simulink library "LiBatteryElements_backup_lib"  (R2020b)
settings: Solver=VariableStepAuto  StartTime=0.0  StopTime=10.0  RelTol=1e-3
values from neighbouring files (symbols this model uses):
  Q = capacity*3600*num_cells    [main.m]    (also in main_1S2P.m; main_cell.m = 4.6)
  SOC_0 = 1    [main.m]    (also in main_1S2P.m; main_cell.m)
undefined symbols (not defined in the file or in its folder): gcbh, simscape, T_init
libraries: fl_lib x10, $bdroot x4
settings Model: Creator=Vivian  LastModifiedBy=Vivian

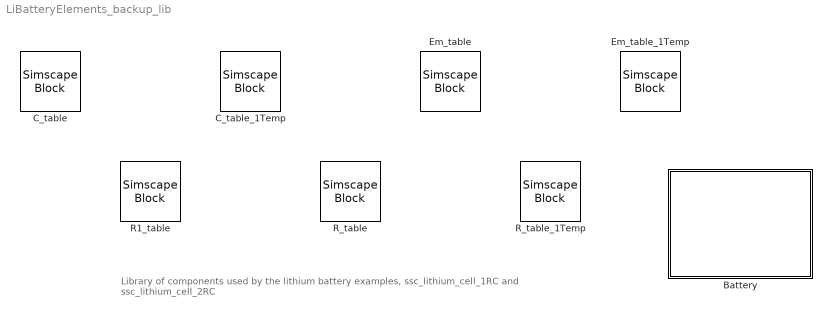
== system LiBatteryElements_backup_lib ==
  note: Library of components used by the lithium battery examples, ssc_lithium_cell_1RC and ssc_lithium_cell_2RC
  Battery : Subsystem
  C_table : SimscapeBlock  DialogController=NetworkEngine.DynNeDlgSource  LoadFcn=simscape.compiler.sli.internal.callback('LoadFcn',gcbh);  SourceFile=LiBatteryElements.C_table  mask(C_table){ComponentPath=LiBatteryElements.C_table, ComponentVariants=["LiBatteryElements.C_table"], ComponentVariantNames=["C_table"], ClassName=C_table, SchemaVersion=1, C_Table=ones(5, 3), C_Table_unit=F, C_Table_conf=compiletime, SOC_Table=[0; .1; .5; .9; 1], SOC_Table_unit=1, SOC_Table_conf=compiletime, Temp_Table=[273.15, 293.15, 313.15], Temp_Table_unit=K, Temp_Table_conf=compiletime, v0=0, v0_unit=V, v0_conf=compiletime}
      mask prompts: C_Table "Matrix of capacitance values, C(SOC,T)"; SOC_Table "State of charge (SOC) breakpoints"; Temp_Table "Temperature (T) breakpoints"; v0 "Initial voltage across capacitor"
      mask help: Models a capacitor where the capacitance value (C) depends on an external physical signal inputs SOC and T. It is assumed that the capacitance value is slowly varying with time, and hence the equation i = C*dv/dt holds.
      mask init:
      | simscape.compiler.sli.internal.preinitmask(gcb);
      settings: CopyFcn=simscape.compiler.sli.internal.callback('CopyFcn',gcbh);  DeleteFcn=simscape.compiler.sli.internal.callback('DeleteFcn',gcbh);  ModelCloseFcn=simscape.compiler.sli.internal.callback('ModelCloseFcn',gcbh);  PreSaveFcn=simscape.compiler.sli.internal.callback('PreSaveFcn',gcbh);  PostSaveFcn=simscape.compiler.sli.internal.callback('PostSaveFcn',gcbh);  PreCopyFcn=simscape.compiler.sli.internal.callback('PreCopyFcn',gcbh);  PreDeleteFcn=simscape.compiler.sli.internal.callback('PreDeleteFcn',gcbh);  InternalSimscapePortConfiguration="{\"Bottom\":[],\"Left\":[{\"id\":\"p\",\"label\":\"+\",\"type\":\"foundation.electrical.electrical\"},{\"id\":\"T\",\"label\":\"T\",\"type\":\"input\"},{\"id\":\"SOC\",\"label\":\"SOC\",\"type\":\"input\"}],\"Right\":[{\"id\":\"n\",\"label\":\"-\",\"type\":\"foundation.electrical.electrical\"}],\"Top\":[]}"
      mask Help: web(nesl_help(gcbh))
      mask TypeOptions C_Table_unit: F | pF | nF | uF | mF
      mask TypeOptions C_Table_conf: compiletime | runtime
      mask TypeOptions SOC_Table_unit: 1
      mask TypeOptions SOC_Table_conf: compiletime | runtime
      mask TypeOptions Temp_Table_unit: K | degC | degF | degR | deltaK | deltadegC | deltadegF | deltadegR
      mask TypeOptions Temp_Table_conf: compiletime | runtime
      mask TypeOptions v0_unit: V | mV | kV
      mask TypeOptions v0_conf: compiletime | runtime
  C_table_1Temp : SimscapeBlock  DialogController=NetworkEngine.DynNeDlgSource  LoadFcn=simscape.compiler.sli.internal.callback('LoadFcn',gcbh);  SourceFile=LiBatteryElements.C_table_1Temp  mask(C_table_1Temp){ComponentPath=LiBatteryElements.C_table_1Temp, ComponentVariants=["LiBatteryElements.C_table_1Temp"], ComponentVariantNames=["C_table_1Temp"], ClassName=C_table_1Temp, SchemaVersion=1, C_Table=ones(5, 1), C_Table_unit=F, C_Table_conf=compiletime, SOC_Table=[0; .1; .5; .9; 1], SOC_Table_unit=1, SOC_Table_conf=compiletime, v0=0, v0_unit=V, v0_conf=compiletime}
      mask prompts: C_Table "Vector of capacitance values"; SOC_Table "Corresponding SOC breakpoints"; v0 "Initial voltage across capacitor"
      mask help: Models a capacitor where the capacitance value (C) depends on an external physical signal input SOC. It is assumed that the capacitance value is slowly varying with time, and hence the equation i = C*dv/dt holds.
      mask init:
      | simscape.compiler.sli.internal.preinitmask(gcb);
      settings: CopyFcn=simscape.compiler.sli.internal.callback('CopyFcn',gcbh);  DeleteFcn=simscape.compiler.sli.internal.callback('DeleteFcn',gcbh);  ModelCloseFcn=simscape.compiler.sli.internal.callback('ModelCloseFcn',gcbh);  PreSaveFcn=simscape.compiler.sli.internal.callback('PreSaveFcn',gcbh);  PostSaveFcn=simscape.compiler.sli.internal.callback('PostSaveFcn',gcbh);  PreCopyFcn=simscape.compiler.sli.internal.callback('PreCopyFcn',gcbh);  PreDeleteFcn=simscape.compiler.sli.internal.callback('PreDeleteFcn',gcbh);  InternalSimscapePortConfiguration="{\"Bottom\":[],\"Left\":[{\"id\":\"p\",\"label\":\"+\",\"type\":\"foundation.electrical.electrical\"},{\"id\":\"SOC\",\"label\":\"SOC\",\"type\":\"input\"}],\"Right\":[{\"id\":\"n\",\"label\":\"-\",\"type\":\"foundation.electrical.electrical\"}],\"Top\":[]}"
      mask Help: web(nesl_help(gcbh))
      mask TypeOptions C_Table_unit: F | pF | nF | uF | mF
      mask TypeOptions C_Table_conf: compiletime | runtime
      mask TypeOptions SOC_Table_unit: 1
      mask TypeOptions SOC_Table_conf: compiletime | runtime
      mask TypeOptions v0_unit: V | mV | kV
      mask TypeOptions v0_conf: compiletime | runtime
  Em_table : SimscapeBlock  DialogController=NetworkEngine.DynNeDlgSource  LoadFcn=simscape.compiler.sli.internal.callback('LoadFcn',gcbh);  SourceFile=LiBatteryElements.Em_table  mask(Em_table){ComponentPath=LiBatteryElements.Em_table, ComponentVariants=["LiBatteryElements.Em_table"], ComponentVariantNames=["Em_table"], ClassName=Em_table, SchemaVersion=1, C_Table=[29, 30, 31], C_Table_unit=hr*A, C_Table_conf=compiletime, Em_Table=3.8 * ones(5, 3), Em_Table_unit=V, Em_Table_conf=compiletime, SOC_Table=[0; .1; .5; .9; 1], SOC_Table_unit=1, SOC_Table_conf=compiletime, Temp_Table=[273.15, 293.15, 313.15], Temp_Table_unit=K, Temp_Table_conf=compiletime, Qinit=0, Qinit_unit=hr*A, Qinit_conf=compiletime}
      mask prompts: C_Table "Capacity values at specified temperature breakpoints"; Em_Table "Matrix of voltage values, Em(SOC,T)"; SOC_Table "State of charge (SOC) breakpoints"; Temp_Table "Temperature (T) breakpoints"; Qinit "Initial charge deficit"
      mask help: This block implements the cell's main branch voltage source, and determines values for capacity (C) and state of charge (SOC). The defining equations depend on cell temperature, T.
      mask init:
      | simscape.compiler.sli.internal.preinitmask(gcb);
      settings: CopyFcn=simscape.compiler.sli.internal.callback('CopyFcn',gcbh);  DeleteFcn=simscape.compiler.sli.internal.callback('DeleteFcn',gcbh);  ModelCloseFcn=simscape.compiler.sli.internal.callback('ModelCloseFcn',gcbh);  PreSaveFcn=simscape.compiler.sli.internal.callback('PreSaveFcn',gcbh);  PostSaveFcn=simscape.compiler.sli.internal.callback('PostSaveFcn',gcbh);  PreCopyFcn=simscape.compiler.sli.internal.callback('PreCopyFcn',gcbh);  PreDeleteFcn=simscape.compiler.sli.internal.callback('PreDeleteFcn',gcbh);  InternalSimscapePortConfiguration="{\"Bottom\":[],\"Left\":[{\"id\":\"p\",\"label\":\"+\",\"type\":\"foundation.electrical.electrical\"},{\"id\":\"C\",\"label\":\"C\",\"type\":\"output\"},{\"id\":\"SOC\",\"label\":\"SOC\",\"type\":\"output\"}],\"Right\":[{\"id\":\"n\",\"label\":\"-\",\"type\":\"foundation.electrical.electrical\"},{\"id\":\"T\",\"label\":\"T\",\"type\":\"input\"}],\"Top\":[]}"
      mask Help: web(nesl_help(gcbh))
      mask TypeOptions C_Table_unit: C | hr*A
      mask TypeOptions C_Table_conf: compiletime | runtime
      mask TypeOptions Em_Table_unit: V | mV | kV
      mask TypeOptions Em_Table_conf: compiletime | runtime
      mask TypeOptions SOC_Table_unit: 1
      mask TypeOptions SOC_Table_conf: compiletime | runtime
      mask TypeOptions Temp_Table_unit: K | degC | degF | degR | deltaK | deltadegC | deltadegF | deltadegR
      mask TypeOptions Temp_Table_conf: compiletime | runtime
      mask TypeOptions Qinit_unit: C | hr*A
      mask TypeOptions Qinit_conf: compiletime | runtime
  Em_table_1Temp : SimscapeBlock  DialogController=NetworkEngine.DynNeDlgSource  LoadFcn=simscape.compiler.sli.internal.callback('LoadFcn',gcbh);  SourceFile=LiBatteryElements.Em_table_1Temp  mask(Em_table_1Temp){ComponentPath=LiBatteryElements.Em_table_1Temp, ComponentVariants=["LiBatteryElements.Em_table_1Temp"], ComponentVariantNames=["Em_table_1Temp"], ClassName=Em_table_1Temp, SchemaVersion=1, Em_Table=3.8 * ones(5, 1), Em_Table_unit=V, Em_Table_conf=compiletime, SOC_Table=[0; .1; .5; .9; 1], SOC_Table_unit=1, SOC_Table_conf=compiletime, C=30, C_unit=hr*A, C_conf=compiletime, Qinit=0, Qinit_unit=hr*A, Qinit_conf=compiletime}
      mask prompts: Em_Table "Vector of voltage values, Em"; SOC_Table "Corresponding SOC breakpoints"; C "Capacity (scalar)"; Qinit "Initial charge deficit"
      mask help: This block implements the main branch voltage source, capacity, and state of charge (SOC). The defining equations are assumed not to depend on temperature.
      mask init:
      | simscape.compiler.sli.internal.preinitmask(gcb);
      settings: CopyFcn=simscape.compiler.sli.internal.callback('CopyFcn',gcbh);  DeleteFcn=simscape.compiler.sli.internal.callback('DeleteFcn',gcbh);  ModelCloseFcn=simscape.compiler.sli.internal.callback('ModelCloseFcn',gcbh);  PreSaveFcn=simscape.compiler.sli.internal.callback('PreSaveFcn',gcbh);  PostSaveFcn=simscape.compiler.sli.internal.callback('PostSaveFcn',gcbh);  PreCopyFcn=simscape.compiler.sli.internal.callback('PreCopyFcn',gcbh);  PreDeleteFcn=simscape.compiler.sli.internal.callback('PreDeleteFcn',gcbh);  InternalSimscapePortConfiguration="{\"Bottom\":[],\"Left\":[{\"id\":\"p\",\"label\":\"+\",\"type\":\"foundation.electrical.electrical\"},{\"id\":\"SOC\",\"label\":\"SOC\",\"type\":\"output\"}],\"Right\":[{\"id\":\"n\",\"label\":\"-\",\"type\":\"foundation.electrical.electrical\"}],\"Top\":[]}"
      mask Help: web(nesl_help(gcbh))
      mask TypeOptions Em_Table_unit: V | mV | kV
      mask TypeOptions Em_Table_conf: compiletime | runtime
      mask TypeOptions SOC_Table_unit: 1
      mask TypeOptions SOC_Table_conf: compiletime | runtime
      mask TypeOptions C_unit: C | hr*A
      mask TypeOptions C_conf: compiletime | runtime
      mask TypeOptions Qinit_unit: C | hr*A
      mask TypeOptions Qinit_conf: compiletime | runtime
  R1_table : SimscapeBlock  DialogController=NetworkEngine.DynNeDlgSource  LoadFcn=simscape.compiler.sli.internal.callback('LoadFcn',gcbh);  SourceFile=LiBatteryElements.R1_table  mask(R1_table){ComponentPath=LiBatteryElements.R1_table, ComponentVariants=["LiBatteryElements.R1_table"], ComponentVariantNames=["R1_table"], ClassName=R1_table, SchemaVersion=1, R_Table=1e-3 * ones(5, 3), R_Table_unit=Ohm, R_Table_conf=compiletime, SOC_Table=[0; .1; .5; .9; 1], SOC_Table_unit=1, SOC_Table_conf=compiletime, Temp_Table=[273.15, 293.15, 313.15], Temp_Table_unit=K, Temp_Table_conf=compiletime}
      mask prompts: R_Table "Matrix of resistance values, R(SOC,T)"; SOC_Table "State of charge (SOC) breakpoints"; Temp_Table "Temperature (T) breakpoints"
      mask help: Models a resistor where the resistance value (R) depends on an external physical signal inputs SOC and T.
      mask init:
      | simscape.compiler.sli.internal.preinitmask(gcb);
      settings: CopyFcn=simscape.compiler.sli.internal.callback('CopyFcn',gcbh);  DeleteFcn=simscape.compiler.sli.internal.callback('DeleteFcn',gcbh);  ModelCloseFcn=simscape.compiler.sli.internal.callback('ModelCloseFcn',gcbh);  PreSaveFcn=simscape.compiler.sli.internal.callback('PreSaveFcn',gcbh);  PostSaveFcn=simscape.compiler.sli.internal.callback('PostSaveFcn',gcbh);  PreCopyFcn=simscape.compiler.sli.internal.callback('PreCopyFcn',gcbh);  PreDeleteFcn=simscape.compiler.sli.internal.callback('PreDeleteFcn',gcbh);  InternalSimscapePortConfiguration="{\"Bottom\":[],\"Left\":[{\"id\":\"p\",\"label\":\"+\",\"type\":\"foundation.electrical.electrical\"},{\"id\":\"T\",\"label\":\"T\",\"type\":\"input\"},{\"id\":\"SOC\",\"label\":\"SOC\",\"type\":\"input\"}],\"Right\":[{\"id\":\"n\",\"label\":\"-\",\"type\":\"foundation.electrical.electrical\"},{\"id\":\"pow\",\"label\":\"POW\",\"type\":\"output\"}],\"Top\":[]}"
      mask Help: web(nesl_help(gcbh))
      mask TypeOptions R_Table_unit: Ohm | kOhm | MOhm | GOhm
      mask TypeOptions R_Table_conf: compiletime | runtime
      mask TypeOptions SOC_Table_unit: 1
      mask TypeOptions SOC_Table_conf: compiletime | runtime
      mask TypeOptions Temp_Table_unit: K | degC | degF | degR | deltaK | deltadegC | deltadegF | deltadegR
      mask TypeOptions Temp_Table_conf: compiletime | runtime
  R_table : SimscapeBlock  DialogController=NetworkEngine.DynNeDlgSource  LoadFcn=simscape.compiler.sli.internal.callback('LoadFcn',gcbh);  SourceFile=LiBatteryElements.R_table  mask(R_table){ComponentPath=LiBatteryElements.R_table, ComponentVariants=["LiBatteryElements.R_table"], ComponentVariantNames=["R_table"], ClassName=R_table, SchemaVersion=1, R_Table=1e-3 * ones(5, 3), R_Table_unit=Ohm, R_Table_conf=compiletime, SOC_Table=[0; .1; .5; .9; 1], SOC_Table_unit=1, SOC_Table_conf=compiletime, Temp_Table=[273.15, 293.15, 313.15], Temp_Table_unit=K, Temp_Table_conf=compiletime}
      mask prompts: R_Table "Matrix of resistance values, R(SOC,T)"; SOC_Table "State of charge (SOC) breakpoints"; Temp_Table "Temperature (T) breakpoints"
      mask help: Models a resistor where the resistance value (R) depends on an external physical signal inputs SOC and T.
      mask init:
      | simscape.compiler.sli.internal.preinitmask(gcb);
      settings: CopyFcn=simscape.compiler.sli.internal.callback('CopyFcn',gcbh);  DeleteFcn=simscape.compiler.sli.internal.callback('DeleteFcn',gcbh);  ModelCloseFcn=simscape.compiler.sli.internal.callback('ModelCloseFcn',gcbh);  PreSaveFcn=simscape.compiler.sli.internal.callback('PreSaveFcn',gcbh);  PostSaveFcn=simscape.compiler.sli.internal.callback('PostSaveFcn',gcbh);  PreCopyFcn=simscape.compiler.sli.internal.callback('PreCopyFcn',gcbh);  PreDeleteFcn=simscape.compiler.sli.internal.callback('PreDeleteFcn',gcbh);  InternalSimscapePortConfiguration="{\"Bottom\":[],\"Left\":[{\"id\":\"p\",\"label\":\"+\",\"type\":\"foundation.electrical.electrical\"},{\"id\":\"T\",\"label\":\"T\",\"type\":\"input\"},{\"id\":\"SOC\",\"label\":\"SOC\",\"type\":\"input\"}],\"Right\":[{\"id\":\"n\",\"label\":\"-\",\"type\":\"foundation.electrical.electrical\"},{\"id\":\"pow\",\"label\":\"POW\",\"type\":\"output\"}],\"Top\":[]}"
      mask Help: web(nesl_help(gcbh))
      mask TypeOptions R_Table_unit: Ohm | kOhm | MOhm | GOhm
      mask TypeOptions R_Table_conf: compiletime | runtime
      mask TypeOptions SOC_Table_unit: 1
      mask TypeOptions SOC_Table_conf: compiletime | runtime
      mask TypeOptions Temp_Table_unit: K | degC | degF | degR | deltaK | deltadegC | deltadegF | deltadegR
      mask TypeOptions Temp_Table_conf: compiletime | runtime
  R_table_1Temp : SimscapeBlock  DialogController=NetworkEngine.DynNeDlgSource  LoadFcn=simscape.compiler.sli.internal.callback('LoadFcn',gcbh);  SourceFile=LiBatteryElements.R_table_1Temp  mask(R_table_1Temp){ComponentPath=LiBatteryElements.R_table_1Temp, ComponentVariants=["LiBatteryElements.R_table_1Temp"], ComponentVariantNames=["R_table_1Temp"], ClassName=R_table_1Temp, SchemaVersion=1, R_Table=1e-3 * ones(5, 1), R_Table_unit=Ohm, R_Table_conf=compiletime, SOC_Table=[0; .1; .5; .9; 1], SOC_Table_unit=1, SOC_Table_conf=compiletime}
      mask prompts: R_Table "Vector of resistance values"; SOC_Table "Corresponding SOC breakpoints"
      mask help: Models a resistor where the resistance value (R) depends on an external physical signal input SOC.
      mask init:
      | simscape.compiler.sli.internal.preinitmask(gcb);
      settings: CopyFcn=simscape.compiler.sli.internal.callback('CopyFcn',gcbh);  DeleteFcn=simscape.compiler.sli.internal.callback('DeleteFcn',gcbh);  ModelCloseFcn=simscape.compiler.sli.internal.callback('ModelCloseFcn',gcbh);  PreSaveFcn=simscape.compiler.sli.internal.callback('PreSaveFcn',gcbh);  PostSaveFcn=simscape.compiler.sli.internal.callback('PostSaveFcn',gcbh);  PreCopyFcn=simscape.compiler.sli.internal.callback('PreCopyFcn',gcbh);  PreDeleteFcn=simscape.compiler.sli.internal.callback('PreDeleteFcn',gcbh);  InternalSimscapePortConfiguration="{\"Bottom\":[],\"Left\":[{\"id\":\"p\",\"label\":\"+\",\"type\":\"foundation.electrical.electrical\"},{\"id\":\"SOC\",\"label\":\"SOC\",\"type\":\"input\"}],\"Right\":[{\"id\":\"n\",\"label\":\"-\",\"type\":\"foundation.electrical.electrical\"}],\"Top\":[]}"
      mask Help: web(nesl_help(gcbh))
      mask TypeOptions R_Table_unit: Ohm | kOhm | MOhm | GOhm
      mask TypeOptions R_Table_conf: compiletime | runtime
      mask TypeOptions SOC_Table_unit: 1
      mask TypeOptions SOC_Table_conf: compiletime | runtime

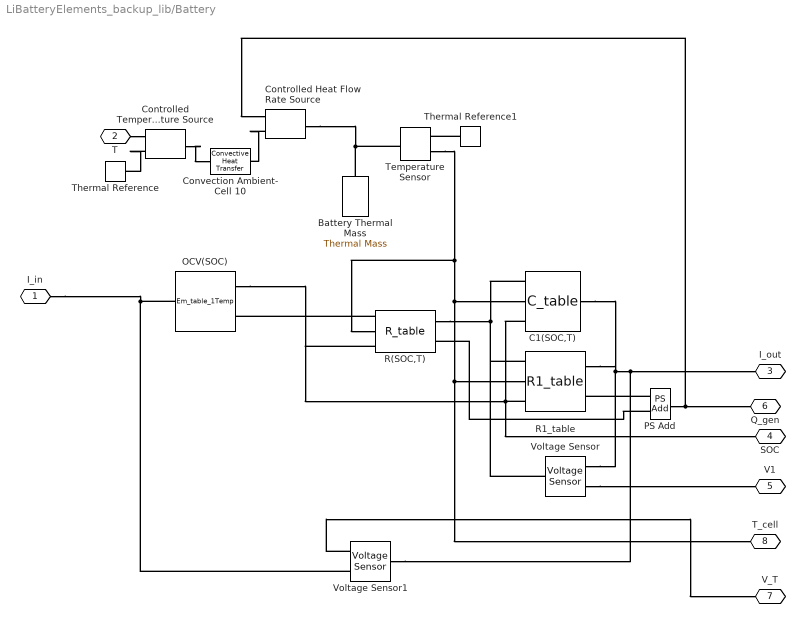
== system LiBatteryElements_backup_lib/Battery ==
  Battery Thermal Mass : fl_lib/Thermal/Thermal Elements/Thermal Mass  mass=cell_mass kg  sp_heat=cell_Cp_heat J/kg/K  T_specify=on  T_priority=High  T=T_init K  T_nominal_specify=off  T_nominal_unit=K  T_nominal_value=1  Q_specify=off  Q_priority=None  Q=0 W  Q_nominal_specify=off  Q_nominal_unit=W  Q_nominal_value=1
      settings: SourceProductName=Foundation Library
  C1(SOC,T) : $bdroot/C_table  C_Table=C1 F  SOC_Table=SOC_RC  Temp_Table=T_RC degC  v0=0 V
      settings: InternalSimscapePortConfiguration="{\"Bottom\":[],\"Left\":[{\"id\":\"p\",\"label\":\"+\",\"type\":\"foundation.electrical.electrical\"},{\"id\":\"T\",\"label\":\"T\",\"type\":\"input\"},{\"id\":\"SOC\",\"label\":\"SOC\",\"type\":\"input\"}],\"Right\":[{\"id\":\"n\",\"label\":\"-\",\"type\":\"foundation.electrical.electrical\"}],\"Top\":[]}"
  Controlled Temperature Source : fl_lib/Thermal/Thermal Sources/Controlled Temperature Source
  Controlled Heat Flow Rate Source : fl_lib/Thermal/Thermal Sources/Controlled Heat Flow Rate Source
      settings: SourceProductName=Foundation Library
  Convection Ambient- Cell 10 : fl_lib/Thermal/Thermal Elements/Convective Heat Transfer  area=cell_area m^2  heat_tr_coeff=h_conv W/(m^2 * K)  T_specify=off  T_priority=None  T=0 K  T_nominal_specify=off  T_nominal_unit=K  T_nominal_value=1  Q_specify=off  Q_priority=None  Q=0 W  Q_nominal_specify=off  Q_nominal_unit=W  Q_nominal_value=1
      settings: SourceProductName=Foundation Library
  OCV(SOC) : $bdroot/Em_table_1Temp  Em_Table=OCV V  SOC_Table=SOC_OCV  C=Q hr*A  Qinit=(1-SOC_0)*Q hr*A
      settings: InternalSimscapePortConfiguration="{\"Bottom\":[],\"Left\":[{\"id\":\"p\",\"label\":\"+\",\"type\":\"foundation.electrical.electrical\"},{\"id\":\"SOC\",\"label\":\"SOC\",\"type\":\"output\"}],\"Right\":[{\"id\":\"n\",\"label\":\"-\",\"type\":\"foundation.electrical.electrical\"}],\"Top\":[]}"
  PS Add : fl_lib/Physical Signals/Functions/PS Add
  R(SOC,T) : $bdroot/R_table  R_Table=Rs Ohm  SOC_Table=SOC_RC  Temp_Table=T_RC degC
      settings: InternalSimscapePortConfiguration="{\"Bottom\":[],\"Left\":[{\"id\":\"p\",\"label\":\"+\",\"type\":\"foundation.electrical.electrical\"},{\"id\":\"T\",\"label\":\"T\",\"type\":\"input\"},{\"id\":\"SOC\",\"label\":\"SOC\",\"type\":\"input\"}],\"Right\":[{\"id\":\"n\",\"label\":\"-\",\"type\":\"foundation.electrical.electrical\"},{\"id\":\"pow\",\"label\":\"POW\",\"type\":\"output\"}],\"Top\":[]}"
  R1_table : $bdroot/R1_table  R_Table=R1 Ohm  SOC_Table=SOC_RC  Temp_Table=T_RC K
      settings: InternalSimscapePortConfiguration="{\"Bottom\":[],\"Left\":[{\"id\":\"p\",\"label\":\"+\",\"type\":\"foundation.electrical.electrical\"},{\"id\":\"T\",\"label\":\"T\",\"type\":\"input\"},{\"id\":\"SOC\",\"label\":\"SOC\",\"type\":\"input\"}],\"Right\":[{\"id\":\"n\",\"label\":\"-\",\"type\":\"foundation.electrical.electrical\"},{\"id\":\"pow\",\"label\":\"POW\",\"type\":\"output\"}],\"Top\":[]}"
  Temperature Sensor : fl_lib/Thermal/Thermal Sensors/Temperature Sensor
      settings: SourceProductName=Foundation Library
  Thermal Reference : fl_lib/Thermal/Thermal Elements/Thermal Reference
  Thermal Reference1 : fl_lib/Thermal/Thermal Elements/Thermal Reference
      settings: SourceProductName=Foundation Library
  Voltage Sensor : fl_lib/Electrical/Electrical Sensors/Voltage Sensor
  Voltage Sensor1 : fl_lib/Electrical/Electrical Sensors/Voltage Sensor
  I_in : PMIOPort  Side=Left
  T : PMIOPort  Port=2  Side=Left
  I_out : PMIOPort  Port=3  Side=Right
  SOC : PMIOPort  Port=4  Side=Right
  V1 : PMIOPort  Port=5  Side=Right
  Q_gen : PMIOPort  Port=6  Side=Right
  V_T : PMIOPort  Port=7  Side=Right
  T_cell : PMIOPort  Port=8  Side=Right
  connections:
  Voltage Sensor/LConn1 -- R1_table/LConn1 -- C1(SOC,T)/LConn1 -- R(SOC,T)/RConn1
  Voltage Sensor/RConn2 -- R1_table/RConn1 -- C1(SOC,T)/RConn1 -- Voltage Sensor1/LConn1 -- I_out/RConn1
  R(SOC,T)/LConn1 -- OCV(SOC)/LConn1
  PS Add/RConn1 -- Controlled Heat Flow Rate Source/RConn1 -- Q_gen/RConn1
  I_in/RConn1 -- Voltage Sensor1/RConn2 -- OCV(SOC)/RConn1
  R(SOC,T)/LConn3 -- OCV(SOC)/LConn2 -- R1_table/LConn3 -- C1(SOC,T)/LConn3 -- SOC/RConn1
  PS Add/LConn1 -- R1_table/RConn2
  Voltage Sensor1/RConn1 -- V_T/RConn1
  Voltage Sensor/RConn1 -- V1/RConn1
  PS Add/LConn2 -- R(SOC,T)/RConn2
  T/RConn1 -- Controlled Temperature Source/RConn1
  Controlled Temperature Source/RConn2 -- Thermal Reference/LConn1
  Controlled Heat Flow Rate Source/LConn1 -- Battery Thermal Mass/LConn1 -- Temperature Sensor/LConn1
  Controlled Heat Flow Rate Source/RConn2 -- Convection Ambient- Cell 10/RConn1
  Thermal Reference1/LConn1 -- Temperature Sensor/RConn1
  Temperature Sensor/RConn2 -- C1(SOC,T)/LConn2 -- R1_table/LConn2 -- T_cell/RConn1 -- R(SOC,T)/LConn2
  Controlled Temperature Source/LConn1 -- Convection Ambient- Cell 10/LConn1
